simulink model "FractionalOCVoltage"  (R2014a)
settings: Solver=ode3  StartTime=0.0  StopTime=1  MaxStep=0.1  RelTol=1e-3
PreLoadFcn:
  | Ts = 1e-6;
  | G = 1000;
  | PVCellIsc = 7;
  | PVCellVoc = 0.64;
  | PVCellRs = 0.001;
  | tau = 1e-4;
libraries: simulink x1
settings Model: Creator=cosorio  LastModifiedBy=cosorio
settings DataIOCC: LimitDataPoints=off  SignalLoggingSaveFormat=ModelDataLogs  SaveOutput=off  SignalLogging=off  DSMLogging=off  SaveTime=off  OutputTimes=[0]
settings OptimizationCC: InlineParams=on  ExpressionDepthLimit=2147483647
settings DebuggingCC: UnderspecifiedInitializationDetection=Classic  SolverPrmCheckMsg=none  FcnCallInpInsideContextMsg=UseLocalSettings  StateNameClashWarn=warning
settings GRTTargetCC: CombineOutputUpdateFcns=off  GRTInterface=on

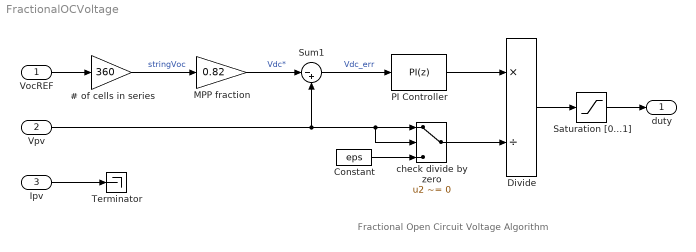
== system FractionalOCVoltage ==
  note: Fractional Open Circuit Voltage Algorithm
  VocREF : Inport  OutDataTypeStr=double  PortDimensions=1  SampleTime=[0.0001,0]
  Vpv : Inport  Port=2  OutDataTypeStr=double  PortDimensions=1  SampleTime=[0.0001,0]
  Ipv : Inport  Port=3  OutDataTypeStr=double  PortDimensions=1  SampleTime=[0.0001,0]
  # of cells in series : Gain  Gain=360
  Constant : Constant  Value=eps
  Divide : Product  Inputs=*/
  MPP fraction : Gain  Gain=0.82
  PI Controller : simulink/Continuous/PID Controller  Controller=PI  TimeDomain=Discrete-time  SampleTime=1e-4  IntegratorMethod=Forward Euler  FilterMethod=Forward Euler  Form=Parallel  P=1  I=250  D=0  N=100  InitialConditionSource=internal  InitialConditionForIntegrator=186.4  InitialConditionForFilter=0  ExternalReset=none  ZeroCross=off  LimitOutput=off  UpperSaturationLimit=1  LowerSaturationLimit=0  LinearizeAsGain=off  AntiWindupMode=none  Kb=1  TrackingMode=off  Kt=1  PParamMin=[]  PParamMax=[]  IParamMin=[]  IParamMax=[]  DParamMin=[]  DParamMax=[]  NParamMin=[]  NParamMax=[]  KbParamMin=[]  KbParamMax=[]  KtParamMin=[]  KtParamMax=[]  POutMin=[]  POutMax=[]  IOutMin=[]  IOutMax=[]  DOutMin=[]  DOutMax=[]  NOutMin=[]  NOutMax=[]  KbOutMin=[]  KbOutMax=[]  KtOutMin=[]  KtOutMax=[]  IntegratorOutMin=[]  IntegratorOutMax=[]  FilterOutMin=[]  FilterOutMax=[]  SumOutMin=[]  SumOutMax=[]  SumI1OutMin=[]  SumI1OutMax=[]  SumI2OutMin=[]  SumI2OutMax=[]  SumI3OutMin=[]  SumI3OutMax=[]  SumDOutMin=[]  SumDOutMax=[]  SaturationOutMin=[]  SaturationOutMax=[]  IntegratorContinuousStateAttributes=''  IntegratorStateMustResolveToSignalObject=off  IntegratorRTWStateStorageClass=Auto  FilterContinuousStateAttributes=''  FilterStateMustResolveToSignalObject=off  FilterRTWStateStorageClass=Auto
  Saturation [0...1] : Saturate  UpperLimit=1  LowerLimit=0
  Sum1 : Sum  Inputs=|-+
  Terminator : Terminator
  check divide by zero : Switch  Criteria=u2 ~= 0
  duty : Outport  OutDataTypeStr=double  PortDimensions=1  SampleTime=[0.0001,0]
  wires:
  Ipv/1 -> Terminator/1
  Saturation [0...1]/1 -> duty/1
  VocREF/1 -> # of cells in series/1
  Divide/1 -> Saturation [0...1]/1
  PI Controller/1 -> Divide/1
  # of cells in series/1 -> MPP fraction/1  "stringVoc"
  MPP fraction/1 -> Sum1/1  "Vdc*"
  Sum1/1 -> PI Controller/1  "Vdc_err"
  Vpv/1 -> check divide by zero/2, check divide by zero/1, Sum1/2
  check divide by zero/1 -> Divide/2
  Constant/1 -> check divide by zero/3
